simulink library "Custom_Valve_Variants_Lib"  (R2022a)
settings: Solver=ode45  StartTime=0.0  StopTime=10.0  RelTol=1e-3
libraries: fl_lib x56, sh_lib x10, Custom_Valve_Orifices_Lib x9, nesl_utility x8, fl_ps_legacy_lib x1
(part 2 of 2)

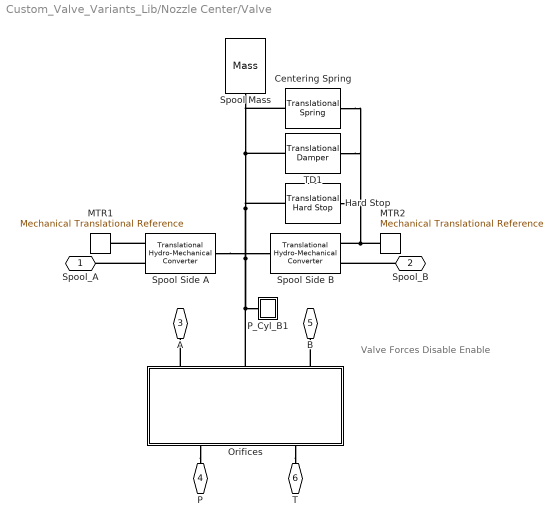
== system Custom_Valve_Variants_Lib/Nozzle Center/Valve ==
  note: Valve Forces
      | Disable Enable
  Centering Spring : fl_lib/Mechanical/Translational Elements/Translational Spring  Tag=Factory Generic  spr_rate=ctr_spr_stiffness N/m  v_specify=off  v_priority=High  v=0 m/s  v_nominal_specify=off  v_nominal_unit=m/s  v_nominal_value=1  f_specify=off  f_priority=High  f=0 N  f_nominal_specify=off  f_nominal_unit=N  f_nominal_value=1  x_specify=on  x_priority=High  x=0 m  x_nominal_specify=off  x_nominal_unit=m  x_nominal_value=1
      settings: SourceProductBaseCode=PW,SS,VE
  Hard Stop : fl_lib/Mechanical/Translational Elements/Translational Hard Stop  Tag=Factory Generic  upper_bnd=max_spool_travel m  lower_bnd=-max_spool_travel m  stiff_up=1e+06 N/m  stiff_low=1e+06 N/m  D_up=150 N/(m/s)  D_low=150 N/(m/s)  model=3  transition=0.1 mm  v_specify=off  v_priority=High  v=0 m/s  v_nominal_specify=off  v_nominal_unit=m/s  v_nominal_value=1  f_specify=off  f_priority=High  f=0 N  f_nominal_specify=off  f_nominal_unit=N  f_nominal_value=1  x_specify=on  x_priority=High  x=0 m  x_nominal_specify=off  x_nominal_unit=m  x_nominal_value=1
      settings: SourceProductBaseCode=PW,SS,VE
  MTR1 : fl_lib/Mechanical/Translational Elements/Mechanical Translational Reference  Tag=Factory Generic
      settings: SourceProductBaseCode=PW,SS,VE
  MTR2 : fl_lib/Mechanical/Translational Elements/Mechanical Translational Reference  Tag=Factory Generic
      settings: SourceProductBaseCode=PW,SS,VE
  Orifices : Subsystem  Variant=on  VariantControlMode=label  LabelModeActiveChoice=No_Force
      settings: AttributesFormatString=%<ActiveVariant>
      mask Display:
      | blk = find_system(gcbh, 'SearchDepth', 1,'LookUnderMasks','on', 'Parent', gcb, 'VariantObject', get_param(gcb,'activevariant'));
      | eval(get_param(blk, 'MaskDisplay'));
  P_Cyl_B1 : Subsystem
  Spool Mass : fl_lib/Mechanical/Translational Elements/Mass  Tag=Factory Generic  mass=spool_mass kg  num_ports=foundation.enum.numPorts2.one  v_specify=on  v_priority=High  v=0 m/s  v_nominal_specify=off  v_nominal_unit=m/s  v_nominal_value=1  f_specify=off  f_priority=High  f=0 N  f_nominal_specify=off  f_nominal_unit=N  f_nominal_value=1
      settings: SourceProductBaseCode=PW,SS,VE
  Spool Side A : fl_lib/Hydraulic/Hydraulic Elements/Translational Hydro-Mechanical Converter  Tag=Factory Generic  area=78 mm^2  or=1  compressibility=0  displacement_spec=foundation.enum.DisplacementSpec.Calculate  init_pos=0 m  V_dead=1e-4 m^3  k_sh=1.4  initial_pressure=0 Pa
      settings: SourceProductBaseCode=PW,SS,VE  InternalSimscapePortConfiguration="{\"Bottom\":[],\"Left\":[{\"id\":\"C\",\"label\":\"C\",\"type\":\"foundation.mechanical.translational.translational\"},{\"id\":\"A\",\"label\":\"A\",\"type\":\"foundation.hydraulic.hydraulic\"}],\"Right\":[{\"id\":\"R\",\"label\":\"R\",\"type\":\"foundation.mechanical.translational.translational\"}],\"Top\":[]}"
  Spool Side B : fl_lib/Hydraulic/Hydraulic Elements/Translational Hydro-Mechanical Converter  Tag=Factory Generic  area=78 mm^2  or=2  compressibility=0  displacement_spec=foundation.enum.DisplacementSpec.Calculate  init_pos=0 m  V_dead=1e-4 m^3  k_sh=1.4  initial_pressure=0 Pa
      settings: SourceProductBaseCode=PW,SS,VE  InternalSimscapePortConfiguration="{\"Bottom\":[],\"Left\":[{\"id\":\"C\",\"label\":\"C\",\"type\":\"foundation.mechanical.translational.translational\"},{\"id\":\"A\",\"label\":\"A\",\"type\":\"foundation.hydraulic.hydraulic\"}],\"Right\":[{\"id\":\"R\",\"label\":\"R\",\"type\":\"foundation.mechanical.translational.translational\"}],\"Top\":[]}"
  TD1 : fl_lib/Mechanical/Translational Elements/Translational Damper  Tag=Factory Generic  D=spool_damping N/(m/s)  v_specify=off  v_priority=High  v=0 m/s  v_nominal_specify=off  v_nominal_unit=m/s  v_nominal_value=1  f_specify=off  f_priority=High  f=0 N  f_nominal_specify=off  f_nominal_unit=N  f_nominal_value=1
      settings: SourceProductBaseCode=PW,SS,VE
  Spool_A : PMIOPort  Side=Left
  Spool_B : PMIOPort  Port=2  Side=Left
  A : PMIOPort  Port=3  Side=Right
  P : PMIOPort  Port=4  Side=Right
  B : PMIOPort  Port=5  Side=Right
  T : PMIOPort  Port=6  Side=Right
  connections:
  Orifices/LConn2 -- T/RConn1
  Orifices/LConn1 -- P/RConn1
  Orifices/RConn3 -- B/RConn1
  Orifices/RConn1 -- A/RConn1
  P_Cyl_B1/LConn1 -- Orifices/RConn2 -- Spool Side A/RConn1 -- Spool Side B/RConn1 -- Hard Stop/LConn1 -- TD1/LConn1 -- Centering Spring/LConn1 -- Spool Mass/LConn1
  Spool Side A/LConn1 -- MTR1/LConn1
  Spool Side A/LConn2 -- Spool_A/RConn1
  Spool_B/RConn1 -- Spool Side B/LConn2
  Hard Stop/RConn1 -- Centering Spring/RConn1 -- TD1/RConn1 -- Spool Side B/LConn1 -- MTR2/LConn1

== system Custom_Valve_Variants_Lib/Nozzle Feedback/Diagram ==
  Diagram : Subsystem
      mask Display: image(imread('Custom_Valve_Flapper_Nozzle_Feedback_Spring_DIAGRAM.jpg'));

== system Custom_Valve_Variants_Lib/Nozzle Feedback/Displacement ==
  Ideal Translational Motion Sensor : fl_lib/Mechanical/Mechanical Sensors/Ideal Translational Motion Sensor  Tag=Factory Generic  offset=0 m
      settings: SourceProductBaseCode=PW,SS,VE
  MTR3 : fl_lib/Mechanical/Translational Elements/Mechanical Translational Reference  Tag=Factory Generic
      settings: SourceProductBaseCode=PW,SS,VE
  PS-Simulink Converter : nesl_utility/PS-Simulink Converter  PhysicalDomain=network_engine_domain  SubClassName=ps_output  LeftPortType=input  RightPortType=output  PseudoPeriodic=off  Frequencies=[]  VectorFormat=1-D array  Unit=1  AffineConversion=off
      settings: SourceProductBaseCode=SS,PW,VE
  Terminator : Terminator
  Spool : PMIOPort  Side=Left
  Disp : PMIOPort  Port=2  Side=Right
  wires:
  PS-Simulink Converter/1 -> Terminator/1
  connections:
  MTR3/LConn1 -- Ideal Translational Motion Sensor/RConn1
  PS-Simulink Converter/LConn1 -- Ideal Translational Motion Sensor/RConn2
  Spool/RConn1 -- Ideal Translational Motion Sensor/LConn1
  Disp/RConn1 -- Ideal Translational Motion Sensor/RConn3

== system Custom_Valve_Variants_Lib/Nozzle Feedback/Sense_x ==
  Ideal Translational Motion Sensor : fl_lib/Mechanical/Mechanical Sensors/Ideal Translational Motion Sensor  Tag=Factory Generic  offset=0 m
      settings: SourceProductBaseCode=PW,SS,VE
  MTR3 : fl_lib/Mechanical/Translational Elements/Mechanical Translational Reference  Tag=Factory Generic
      settings: SourceProductBaseCode=PW,SS,VE
  PS-Simulink Converter2 : nesl_utility/PS-Simulink Converter  PhysicalDomain=network_engine_domain  SubClassName=ps_output  LeftPortType=input  RightPortType=output  PseudoPeriodic=off  Frequencies=[]  VectorFormat=1-D array  Unit=1  AffineConversion=off
      settings: SourceProductBaseCode=SS,PW,VE
  X : PMIOPort  Side=Left
  tag scope: Flapper_x=global
  wires:
  PS-Simulink Converter2/1 -> [Flapper_x]  "Flapper_Position"
  connections:
  Ideal Translational Motion Sensor/RConn3 -- PS-Simulink Converter2/LConn1
  X/RConn1 -- Ideal Translational Motion Sensor/LConn1
  MTR3/LConn1 -- Ideal Translational Motion Sensor/RConn1

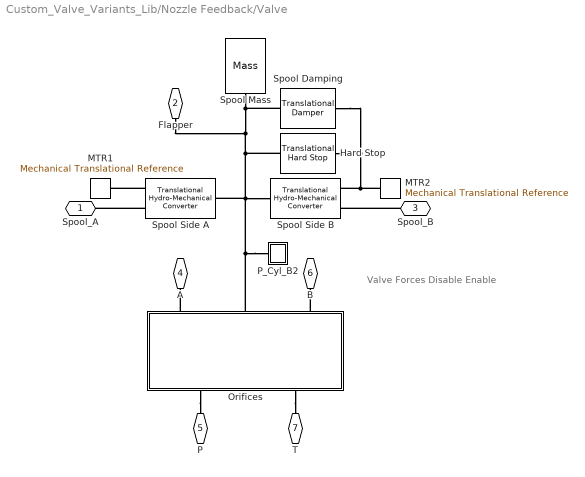
== system Custom_Valve_Variants_Lib/Nozzle Feedback/Valve ==
  note: Valve Forces
      | Disable Enable
  Hard Stop : fl_lib/Mechanical/Translational Elements/Translational Hard Stop  Tag=Factory Generic  upper_bnd=max_spool_travel m  lower_bnd=-max_spool_travel m  stiff_up=1e+06 N/m  stiff_low=1e+06 N/m  D_up=150 N/(m/s)  D_low=150 N/(m/s)  model=3  transition=0.1 mm  v_specify=off  v_priority=High  v=0 m/s  v_nominal_specify=off  v_nominal_unit=m/s  v_nominal_value=1  f_specify=off  f_priority=High  f=0 N  f_nominal_specify=off  f_nominal_unit=N  f_nominal_value=1  x_specify=on  x_priority=High  x=0 m  x_nominal_specify=off  x_nominal_unit=m  x_nominal_value=1
      settings: SourceProductBaseCode=PW,SS,VE
  MTR1 : fl_lib/Mechanical/Translational Elements/Mechanical Translational Reference  Tag=Factory Generic
      settings: SourceProductBaseCode=PW,SS,VE
  MTR2 : fl_lib/Mechanical/Translational Elements/Mechanical Translational Reference  Tag=Factory Generic
      settings: SourceProductBaseCode=PW,SS,VE
  Orifices : Subsystem  Variant=on  VariantControlMode=label  LabelModeActiveChoice=No_Force
      settings: AttributesFormatString=%<ActiveVariant>
      mask Display:
      | blk = find_system(gcbh, 'SearchDepth', 1,'LookUnderMasks','on', 'Parent', gcb, 'VariantObject', get_param(gcb,'activevariant'));
      | eval(get_param(blk, 'MaskDisplay'));
  P_Cyl_B2 : Subsystem
  Spool Damping : fl_lib/Mechanical/Translational Elements/Translational Damper  Tag=Factory Generic  D=spool_damping N/(m/s)  v_specify=off  v_priority=High  v=0 m/s  v_nominal_specify=off  v_nominal_unit=m/s  v_nominal_value=1  f_specify=off  f_priority=High  f=0 N  f_nominal_specify=off  f_nominal_unit=N  f_nominal_value=1
      settings: SourceProductBaseCode=PW,SS,VE
  Spool Mass : fl_lib/Mechanical/Translational Elements/Mass  Tag=Factory Generic  mass=spool_mass kg  num_ports=foundation.enum.numPorts2.one  v_specify=on  v_priority=High  v=0 m/s  v_nominal_specify=off  v_nominal_unit=m/s  v_nominal_value=1  f_specify=off  f_priority=High  f=0 N  f_nominal_specify=off  f_nominal_unit=N  f_nominal_value=1
      settings: SourceProductBaseCode=PW,SS,VE
  Spool Side A : fl_lib/Hydraulic/Hydraulic Elements/Translational Hydro-Mechanical Converter  Tag=Factory Generic  area=78 mm^2  or=1  compressibility=0  displacement_spec=foundation.enum.DisplacementSpec.Calculate  init_pos=0 m  V_dead=1e-4 m^3  k_sh=1.4  initial_pressure=0 Pa
      settings: SourceProductBaseCode=PW,SS,VE  InternalSimscapePortConfiguration="{\"Bottom\":[],\"Left\":[{\"id\":\"C\",\"label\":\"C\",\"type\":\"foundation.mechanical.translational.translational\"},{\"id\":\"A\",\"label\":\"A\",\"type\":\"foundation.hydraulic.hydraulic\"}],\"Right\":[{\"id\":\"R\",\"label\":\"R\",\"type\":\"foundation.mechanical.translational.translational\"}],\"Top\":[]}"
  Spool Side B : fl_lib/Hydraulic/Hydraulic Elements/Translational Hydro-Mechanical Converter  Tag=Factory Generic  area=78 mm^2  or=2  compressibility=0  displacement_spec=foundation.enum.DisplacementSpec.Calculate  init_pos=0 m  V_dead=1e-4 m^3  k_sh=1.4  initial_pressure=0 Pa
      settings: SourceProductBaseCode=PW,SS,VE  InternalSimscapePortConfiguration="{\"Bottom\":[],\"Left\":[{\"id\":\"C\",\"label\":\"C\",\"type\":\"foundation.mechanical.translational.translational\"},{\"id\":\"A\",\"label\":\"A\",\"type\":\"foundation.hydraulic.hydraulic\"}],\"Right\":[{\"id\":\"R\",\"label\":\"R\",\"type\":\"foundation.mechanical.translational.translational\"}],\"Top\":[]}"
  Spool_A : PMIOPort  Side=Left
  Flapper : PMIOPort  Port=2  Side=Left
  Spool_B : PMIOPort  Port=3  Side=Left
  A : PMIOPort  Port=4  Side=Right
  P : PMIOPort  Port=5  Side=Right
  B : PMIOPort  Port=6  Side=Right
  T : PMIOPort  Port=7  Side=Right
  connections:
  Orifices/LConn2 -- T/RConn1
  Orifices/RConn1 -- A/RConn1
  Orifices/LConn1 -- P/RConn1
  Orifices/RConn3 -- B/RConn1
  MTR2/LConn1 -- Hard Stop/RConn1 -- Spool Damping/RConn1 -- Spool Side B/LConn1
  Spool_B/RConn1 -- Spool Side B/LConn2
  Spool Side A/LConn2 -- Spool_A/RConn1
  Spool Side A/LConn1 -- MTR1/LConn1
  P_Cyl_B2/LConn1 -- Orifices/RConn2 -- Spool Side A/RConn1 -- Spool Side B/RConn1 -- Flapper/RConn1 -- Spool Mass/LConn1 -- Spool Damping/LConn1 -- Hard Stop/LConn1

== system Custom_Valve_Variants_Lib/Spool/Diagram ==
  Diagram : Subsystem
      mask Display: image(imread('Custom_Valve_Spool_DIAGRAM.jpg'));

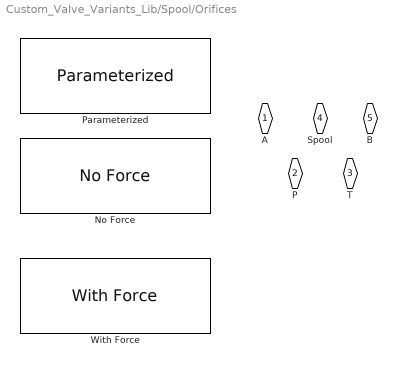
== system Custom_Valve_Variants_Lib/Spool/Orifices ==
  No Force : Custom_Valve_Orifices_Lib/No Force  VariantControl=No_Force  or_width=orifice_width  x0_PA=x0_orifice_PA  x0_PB=x0_orifice_PB  x0_AT=x0_orifice_AT  x0_BT=x0_orifice_BT
  Parameterized : Custom_Valve_Orifices_Lib/Parameterized  VariantControl=Parameterized  or_width=24.5  max_sp_trv=0.005  x0_PA=0  x0_PB=0  x0_AT=0  x0_BT=0
  With Force : Custom_Valve_Orifices_Lib/With Force  VariantControl=With_Force  or_width=orifice_width  x0_PA=x0_orifice_PA  x0_PB=x0_orifice_PB  x0_AT=x0_orifice_AT  x0_BT=x0_orifice_BT  rad_clearance=0.05
  A : PMIOPort  Side=Right
  P : PMIOPort  Port=2  Side=Left
  T : PMIOPort  Port=3  Side=Left
  Spool : PMIOPort  Port=4  Side=Right
  B : PMIOPort  Port=5  Side=Right

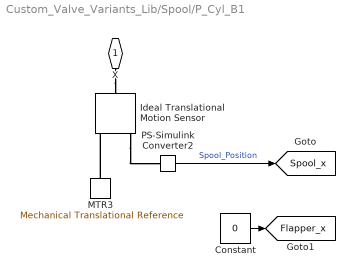
== system Custom_Valve_Variants_Lib/Spool/P_Cyl_B1 ==
  Constant : Constant  Value=0
  Ideal Translational Motion Sensor : fl_lib/Mechanical/Mechanical Sensors/Ideal Translational Motion Sensor  Tag=Factory Generic  offset=0 m
      settings: SourceProductBaseCode=PW,SS,VE
  MTR3 : fl_lib/Mechanical/Translational Elements/Mechanical Translational Reference  Tag=Factory Generic
      settings: SourceProductBaseCode=PW,SS,VE
  PS-Simulink Converter2 : nesl_utility/PS-Simulink Converter  PhysicalDomain=network_engine_domain  SubClassName=ps_output  LeftPortType=input  RightPortType=output  PseudoPeriodic=off  Frequencies=[]  VectorFormat=1-D array  Unit=mm  AffineConversion=off
      settings: SourceProductBaseCode=SS,PW,VE
  X : PMIOPort  Side=Left
  tag scope: Flapper_x=global, Spool_x=global
  wires:
  PS-Simulink Converter2/1 -> [Spool_x]  "Spool_Position"
  Constant/1 -> [Flapper_x]
  connections:
  MTR3/LConn1 -- Ideal Translational Motion Sensor/RConn1
  X/RConn1 -- Ideal Translational Motion Sensor/LConn1
  Ideal Translational Motion Sensor/RConn3 -- PS-Simulink Converter2/LConn1

== system Custom_Valve_Variants_Lib/Nozzle Center/Diagram/Diagram ==

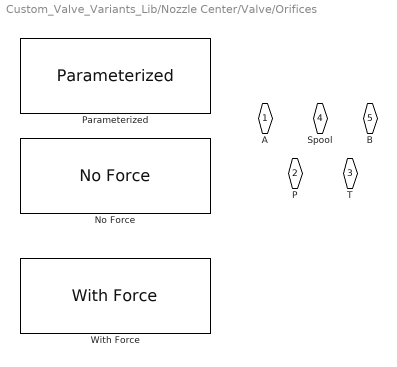
== system Custom_Valve_Variants_Lib/Nozzle Center/Valve/Orifices ==
  No Force : Custom_Valve_Orifices_Lib/No Force  VariantControl=No_Force  or_width=orifice_width  x0_PA=x0_orifice_PA  x0_PB=x0_orifice_PB  x0_AT=x0_orifice_AT  x0_BT=x0_orifice_BT
  Parameterized : Custom_Valve_Orifices_Lib/Parameterized  VariantControl=Parameterized  or_width=24.5  max_sp_trv=0.005  x0_PA=0  x0_PB=0  x0_AT=0  x0_BT=0
  With Force : Custom_Valve_Orifices_Lib/With Force  VariantControl=With_Force  or_width=orifice_width  x0_PA=x0_orifice_PA  x0_PB=x0_orifice_PB  x0_AT=x0_orifice_AT  x0_BT=x0_orifice_BT  rad_clearance=0.05
  A : PMIOPort  Side=Right
  P : PMIOPort  Port=2  Side=Left
  T : PMIOPort  Port=3  Side=Left
  Spool : PMIOPort  Port=4  Side=Right
  B : PMIOPort  Port=5  Side=Right

== system Custom_Valve_Variants_Lib/Nozzle Center/Valve/P_Cyl_B1 ==
  Ideal Translational Motion Sensor : fl_lib/Mechanical/Mechanical Sensors/Ideal Translational Motion Sensor  Tag=Factory Generic  offset=0 m
      settings: SourceProductBaseCode=PW,SS,VE
  MTR3 : fl_lib/Mechanical/Translational Elements/Mechanical Translational Reference  Tag=Factory Generic
      settings: SourceProductBaseCode=PW,SS,VE
  PS-Simulink Converter2 : nesl_utility/PS-Simulink Converter  PhysicalDomain=network_engine_domain  SubClassName=ps_output  LeftPortType=input  RightPortType=output  PseudoPeriodic=off  Frequencies=[]  VectorFormat=1-D array  Unit=mm  AffineConversion=off
      settings: SourceProductBaseCode=SS,PW,VE
  X : PMIOPort  Side=Left
  tag scope: Spool_x=global
  wires:
  PS-Simulink Converter2/1 -> [Spool_x]  "Spool_Position"
  connections:
  Ideal Translational Motion Sensor/RConn3 -- PS-Simulink Converter2/LConn1
  X/RConn1 -- Ideal Translational Motion Sensor/LConn1
  MTR3/LConn1 -- Ideal Translational Motion Sensor/RConn1

== system Custom_Valve_Variants_Lib/Nozzle Feedback/Diagram/Diagram ==

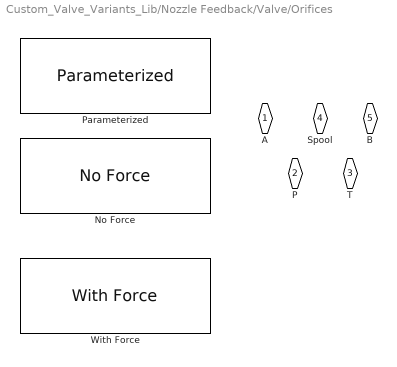
== system Custom_Valve_Variants_Lib/Nozzle Feedback/Valve/Orifices ==
  No Force : Custom_Valve_Orifices_Lib/No Force  VariantControl=No_Force  or_width=orifice_width  x0_PA=x0_orifice_PA  x0_PB=x0_orifice_PB  x0_AT=x0_orifice_AT  x0_BT=x0_orifice_BT
  Parameterized : Custom_Valve_Orifices_Lib/Parameterized  VariantControl=Parameterized  or_width=24.5  max_sp_trv=0.005  x0_PA=0  x0_PB=0  x0_AT=0  x0_BT=0
  With Force : Custom_Valve_Orifices_Lib/With Force  VariantControl=With_Force  or_width=orifice_width  x0_PA=x0_orifice_PA  x0_PB=x0_orifice_PB  x0_AT=x0_orifice_AT  x0_BT=x0_orifice_BT  rad_clearance=0.05
  A : PMIOPort  Side=Right
  P : PMIOPort  Port=2  Side=Left
  T : PMIOPort  Port=3  Side=Left
  Spool : PMIOPort  Port=4  Side=Right
  B : PMIOPort  Port=5  Side=Right

== system Custom_Valve_Variants_Lib/Nozzle Feedback/Valve/P_Cyl_B2 ==
  Ideal Translational Motion Sensor : fl_lib/Mechanical/Mechanical Sensors/Ideal Translational Motion Sensor  Tag=Factory Generic  offset=0 m
      settings: SourceProductBaseCode=PW,SS,VE
  MTR3 : fl_lib/Mechanical/Translational Elements/Mechanical Translational Reference  Tag=Factory Generic
      settings: SourceProductBaseCode=PW,SS,VE
  PS-Simulink Converter2 : nesl_utility/PS-Simulink Converter  PhysicalDomain=network_engine_domain  SubClassName=ps_output  LeftPortType=input  RightPortType=output  PseudoPeriodic=off  Frequencies=[]  VectorFormat=1-D array  Unit=mm  AffineConversion=off
      settings: SourceProductBaseCode=SS,PW,VE
  X : PMIOPort  Side=Left
  tag scope: Spool_x=global
  wires:
  PS-Simulink Converter2/1 -> [Spool_x]  "Spool_Position"
  connections:
  Ideal Translational Motion Sensor/RConn3 -- PS-Simulink Converter2/LConn1
  X/RConn1 -- Ideal Translational Motion Sensor/LConn1
  MTR3/LConn1 -- Ideal Translational Motion Sensor/RConn1

== system Custom_Valve_Variants_Lib/Spool/Diagram/Diagram ==
